simulink library "dlw"  (Simulink 8.1)
settings: Solver=ode1  StartTime=0.0  StopTime=Inf  FixedStep=0.001  RelTol=1e-3
PostLoadFcn:
  | , if any(exist('dsrtsu_mdlpostloadfcn', 'file') == [2, 3, 6]), try dsrtsu_mdlpostloadfcn('Execute', bdroot); catch fprintf('Error in PostLoadFcn (dsrtsu_mdlpostloadfcn) for model "%s":\n %s\n', bdroot, lasterr); end, end,
undefined symbols (not defined in the file or in its folder): AACC_ACCVehSpd_mps, KACC_ACCClearanceToWarn_m, KACC_ACCMinTimeGapToWarn_s, KACC_ACCSpeedToWarn_kph, KACC_ACCTimeGapToWarn_s, MACC_ACCISODeceleration_mps2, ZERO_FLOAT
libraries: hcu_lib x2
settings Model: DSRTSU_INTERNAL_RTI_VER=450  DSRTSU_INTERNAL_RTI_TYPE=rti1401  RTICANMMDATA=struct('GeneralSetupData',struct('modelroot','D:\ELN150201_TAIWAN\trunk\AdasDragon\software\sw_development\arch\app\acc','generalsettings',struct('filesettings',struct('destfolder',struct('Name','RTICANMM_FILES','Check',1),'buildfolder',struct('Name','.','Check',1),'AbsDestfolder',struct('Name','D:\ELN150201_TAIWAN\trunk\AdasDragon\software\sw_development\arch\app\acc\RTICANMM_FILES'),'AbsBuildfolder',struct('Name','D:\ELN150201_TAIWAN\trunk\AdasDragon\software\sw_development\arch\app\acc'))),'options',struct('addpaths',1,'rmpaths',1,'addtrcexclusion',logical(1),'cannavigator',struct('checkmonitoring',0),'show_usrtrc',0,'use_usrtrc',0),'advanced',struct('options',[1 1 1 1 1 1 1 1 1 1 1 1 1 1 1 1 1 1 1 1 1 1 1 1 1 1 1 1 1 1 1 1 1 1 1 1 1 1 1 1 1 1 1 1 1 1 1 1 1 1 1 1 1 1 1 1 1 1 1 1 1 1 1 1 1 1 1 1 1 1 1 1 1 1 1 1 1 1 1 1 1 1 1 1 1 1 1 1 1 1 1 1 1 1 1 1 1 1 1 1]),'MPSetup',{{}},'modelname','dlw','block','dlw'))  DSRTSU_INTERNAL_RTIFPGA=40  Creator=AT015411  LastModifiedBy=AT015555

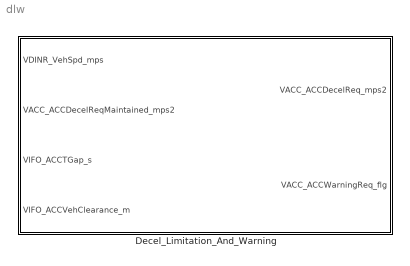
== system dlw ==
  Decel_Limitation_And_Warning : Subsystem

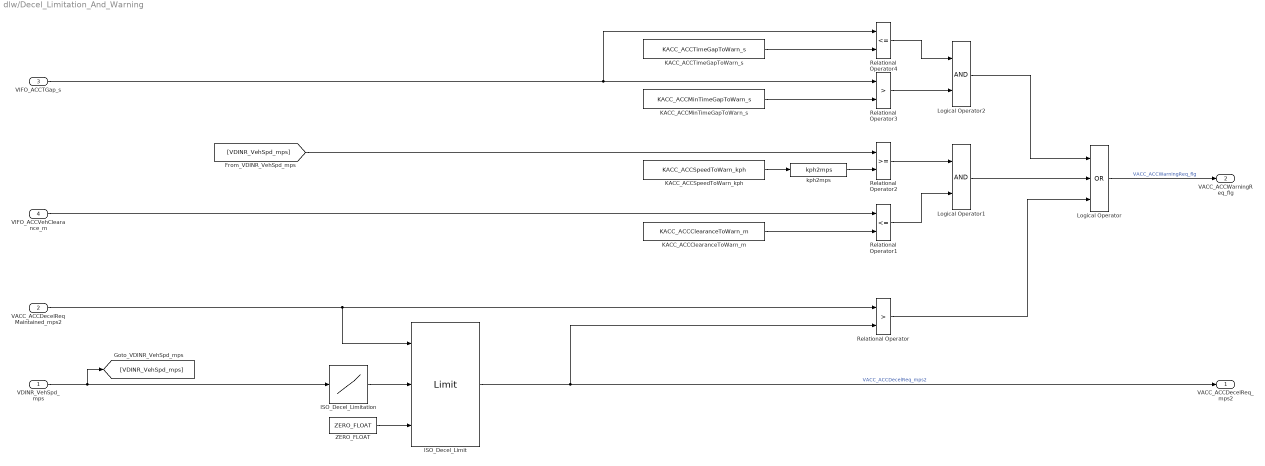
== system dlw/Decel_Limitation_And_Warning ==
  VDINR_VehSpd_mps : Inport
  VACC_ACCDecelReqMaintained_mps2 : Inport  Port=2
  VIFO_ACCTGap_s : Inport  Port=3
  VIFO_ACCVehClearance_m : Inport  Port=4
  ISO_Decel_Limit : hcu_lib/Limit  SystemSampleTime=-1
  ISO_Decel_Limitation : Lookup_n-D  NumberOfTableDimensions=1  BreakpointsForDimension1=AACC_ACCVehSpd_mps  Table=MACC_ACCISODeceleration_mps2  ExtrapMethod=Clip  UseLastTableValue=on  RndMeth=Simplest  InputSameDT=on
  KACC_ACCClearanceToWarn_m : Constant  Value=KACC_ACCClearanceToWarn_m
  KACC_ACCMinTimeGapToWarn_s : Constant  Value=KACC_ACCMinTimeGapToWarn_s
  KACC_ACCSpeedToWarn_kph : Constant  Value=KACC_ACCSpeedToWarn_kph
  KACC_ACCTimeGapToWarn_s : Constant  Value=KACC_ACCTimeGapToWarn_s
  Logical Operator : Logic  Operator=OR  Inputs=3  AllPortsSameDT=off  OutDataTypeStr=boolean
  Logical Operator1 : Logic  AllPortsSameDT=off  OutDataTypeStr=boolean
  Logical Operator2 : Logic  AllPortsSameDT=off  OutDataTypeStr=boolean
  Relational Operator : RelationalOperator  Operator=>  OutDataTypeStr=boolean
  Relational Operator1 : RelationalOperator  Operator=<=  OutDataTypeStr=boolean
  Relational Operator2 : RelationalOperator  OutDataTypeStr=boolean
  Relational Operator3 : RelationalOperator  Operator=>  OutDataTypeStr=boolean
  Relational Operator4 : RelationalOperator  Operator=<=  OutDataTypeStr=boolean
  ZERO_FLOAT : Constant  Value=ZERO_FLOAT
  kph2mps : hcu_lib/kph2mps
  VACC_ACCDecelReq_mps2 : Outport
  VACC_ACCWarningReq_flg : Outport  Port=2
  wires:
  VACC_ACCDecelReqMaintained_mps2/1 -> ISO_Decel_Limit/1, Relational Operator/1
  ISO_Decel_Limitation/1 -> ISO_Decel_Limit/2
  VDINR_VehSpd_mps/1 -> [VDINR_VehSpd_mps], ISO_Decel_Limitation/1
  Logical Operator/1 -> VACC_ACCWarningReq_flg/1  "VACC_ACCWarningReq_flg"
  ZERO_FLOAT/1 -> ISO_Decel_Limit/3
  VIFO_ACCVehClearance_m/1 -> Relational Operator1/1
  Relational Operator1/1 -> Logical Operator1/2
  Relational Operator/1 -> Logical Operator/3
  KACC_ACCClearanceToWarn_m/1 -> Relational Operator1/2
  KACC_ACCSpeedToWarn_kph/1 -> kph2mps/1
  [VDINR_VehSpd_mps] -> Relational Operator2/1
  Relational Operator2/1 -> Logical Operator1/1
  Logical Operator1/1 -> Logical Operator/2
  kph2mps/1 -> Relational Operator2/2
  KACC_ACCTimeGapToWarn_s/1 -> Relational Operator4/2
  VIFO_ACCTGap_s/1 -> Relational Operator4/1, Relational Operator3/1
  ISO_Decel_Limit/1 -> Relational Operator/2, VACC_ACCDecelReq_mps2/1  "VACC_ACCDecelReq_mps2"
  Relational Operator3/1 -> Logical Operator2/2
  Relational Operator4/1 -> Logical Operator2/1
  Logical Operator2/1 -> Logical Operator/1
  KACC_ACCMinTimeGapToWarn_s/1 -> Relational Operator3/2
